simulink model "HeatSelection"  (R2021a)
settings: Solver=VariableStepAuto  StartTime=0.0  StopTime=100.0  RelTol=1e-3
values from neighbouring files (symbols this model uses):
  dif = [1.0 1.0 1.0 1.0]    [InitialInputsGenerate.m]    (also in initializer.m = [1.0 1.0 1.0 10])
  get = [17.0 16.0 16.0 17.0]    [InitialInputsGenerate.m]    (also in initializer.m)
undefined symbols (not defined in the file or in its folder): h1, h2, h3, h4
settings Model: Creator=Kendra  LastModifiedBy=Kendra
settings ModelReferenceCC: UpdateModelReferenceTargets=Force

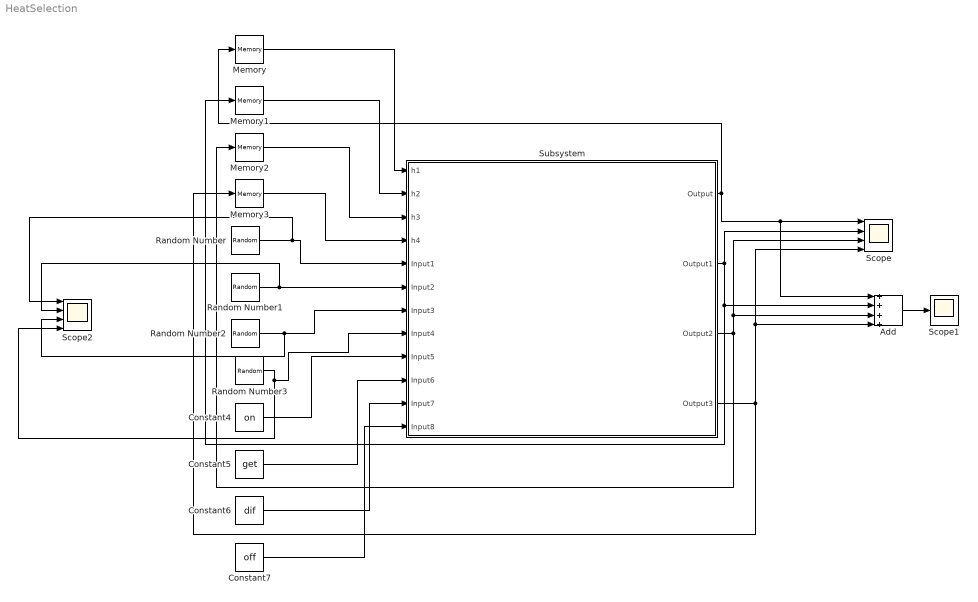
== system HeatSelection ==
  Add : Sum  Inputs=++++
  Constant4 : Constant  Value=on
  Constant5 : Constant  Value=get
  Constant6 : Constant  Value=dif
  Constant7 : Constant  Value=off
  Memory : Memory  InitialCondition=h1  InheritSampleTime=on
  Memory1 : Memory  InitialCondition=h2  InheritSampleTime=on
  Memory2 : Memory  InitialCondition=h3  InheritSampleTime=on
  Memory3 : Memory  InitialCondition=h4  InheritSampleTime=on
  Random Number : RandomNumber  Mean=16.5  SampleTime=1
  Random Number1 : RandomNumber  Mean=16.5  Seed=1  SampleTime=1
  Random Number2 : RandomNumber  Mean=16.5  Seed=2  SampleTime=1
  Random Number3 : RandomNumber  Mean=16.5  Seed=3  SampleTime=1
  Scope : Scope  NumInputPorts=4
  Scope1 : Scope
  Scope2 : Scope  NumInputPorts=4
  Subsystem : Subsystem
  wires:
  Constant5/1 -> Subsystem/10(Input6)
  Random Number1/1 -> Scope2/2, Subsystem/6(Input2)
  Constant6/1 -> Subsystem/11(Input7)
  Subsystem/4(Output3) -> Memory3/1, Add/4, Scope/4
  Memory1/1 -> Subsystem/2("h2 ")
  Subsystem/3(Output2) -> Add/3, Scope/3, Memory2/1
  Memory2/1 -> Subsystem/3("h3 ")
  Constant4/1 -> Subsystem/9(Input5)
  Random Number2/1 -> Scope2/3, Subsystem/7(Input3)
  Memory/1 -> Subsystem/1("h1 ")
  Subsystem/2(Output1) -> Memory1/1, Add/2, Scope/2
  Random Number3/1 -> Scope2/4, Subsystem/8(Input4)
  Subsystem/1(Output) -> Memory/1, Add/1, Scope/1
  Constant7/1 -> Subsystem/12(Input8)
  Random Number/1 -> Scope2/1, Subsystem/5(Input1)
  Add/1 -> Scope1/1
  Memory3/1 -> Subsystem/4(h4)

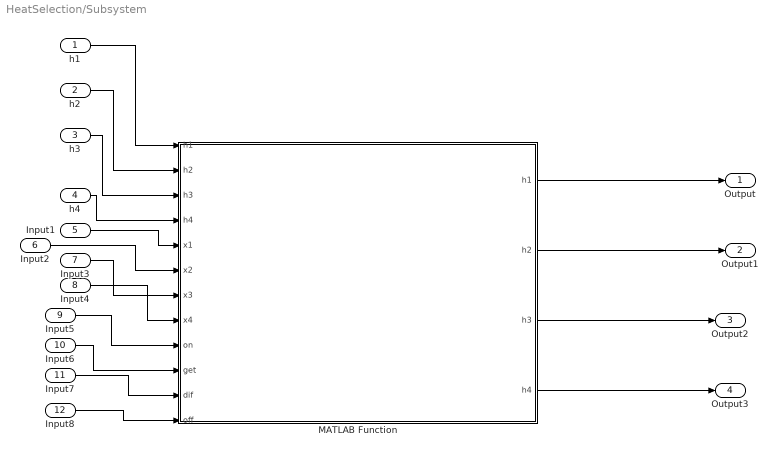
== system HeatSelection/Subsystem ==
  "h1 " : Inport
  "h2 " : Inport  Port=2
  "h3 " : Inport  Port=3
  h4 : Inport  Port=4
  Input1 : Inport  Port=5
  Input2 : Inport  Port=6
  Input3 : Inport  Port=7
  Input4 : Inport  Port=8
  Input5 : Inport  Port=9
  Input6 : Inport  Port=10
  Input7 : Inport  Port=11
  Input8 : Inport  Port=12
  MATLAB Function : MATLAB Function  TreatAsAtomicUnit=on
  Output : Outport
  Output1 : Outport  Port=2
  Output2 : Outport  Port=3
  Output3 : Outport  Port=4
  wires:
  MATLAB Function/2(h2) -> Output1/1
  MATLAB Function/3(h3) -> Output2/1
  MATLAB Function/4(h4) -> Output3/1
  MATLAB Function/1(h1) -> Output/1
  "h1 "/1 -> MATLAB Function/1("h1 ")
  "h2 "/1 -> MATLAB Function/2("h2 ")
  "h3 "/1 -> MATLAB Function/3("h3 ")
  Input1/1 -> MATLAB Function/5(x1)
  Input2/1 -> MATLAB Function/6(x2)
  h4/1 -> MATLAB Function/4("h4 ")
  Input3/1 -> MATLAB Function/7(x3)
  Input4/1 -> MATLAB Function/8(x4)
  Input5/1 -> MATLAB Function/9(on)
  Input6/1 -> MATLAB Function/10(get)
  Input7/1 -> MATLAB Function/11(dif)
  Input8/1 -> MATLAB Function/12(off)

== matlab function HeatSelection/Subsystem/MATLAB Function ==
  data: h1 input; h1 output; h2 input; h3 input; h4 input; x1 input; x2 input; x3 input; x4 input; on input; get input; dif input; off input; h2 output; h3 output; h4 output
function [h1,h2,h3,h4] = SelectHeaters(h1,h2,h3,h4,x1,x2,x3,x4,on,get,dif,off)
x = [x1,x2,x3,x4];
h = [h1,h2,h3,h4];
persistent locations;
hnew = zeros(1,4);
if isempty(locations)
    locations = h;
end
ind = find(locations == 1);

biggestdiff = 0;
newind1 = 1;

for i = 1:1:4
    if x(i) <= get(i) && x(ind(1)) - x(i) >= dif(i)
        curdiff = on(i)-x(i);
        if curdiff > biggestdiff
            biggestdiff = curdiff;
            newind1 = i;
        end
    end
end

locations(newind1) = 1;
if x(newind1) <= on(i) && x(i) < off(i)
    hnew(newind1) = 1;
end

biggestdiff = 0;
newind2 = 1;
for i = 1:1:4
    if x(i) <= get(i) && x(ind(1)) - x(i) >= dif(i) && i ~= newind1
        curdiff = on(i)-x(i);
        if curdiff > biggestdiff
            biggestdiff = curdiff;
            newind2 = i;
        end
    end
end

locations(newind2) = 1;
if x(i) <= on(i) && x(i) < off(i)
    hnew(newind2) = 1;
end

h1 = hnew(1);
h2 = hnew(2);
h3 = hnew(3);
h4 = hnew(4);
